simulink model "Dc_shunt_motor_model_not_verified"  (R2021b)
settings: Solver=VariableStepAuto  StartTime=0.0  StopTime=10.0  RelTol=1e-3
settings Model: Creator=victor  LastModifiedBy=victor

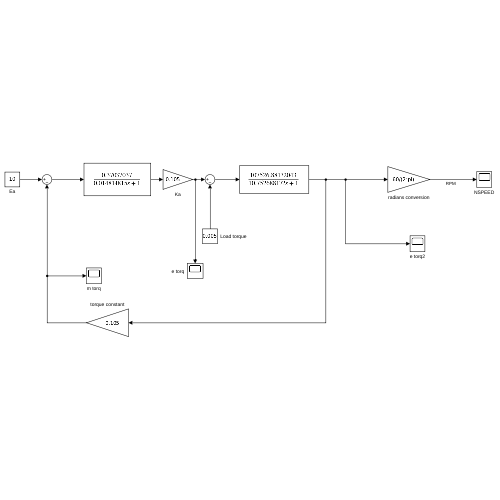
[thumbnail: Simulink's stored preview of the top-level diagram]
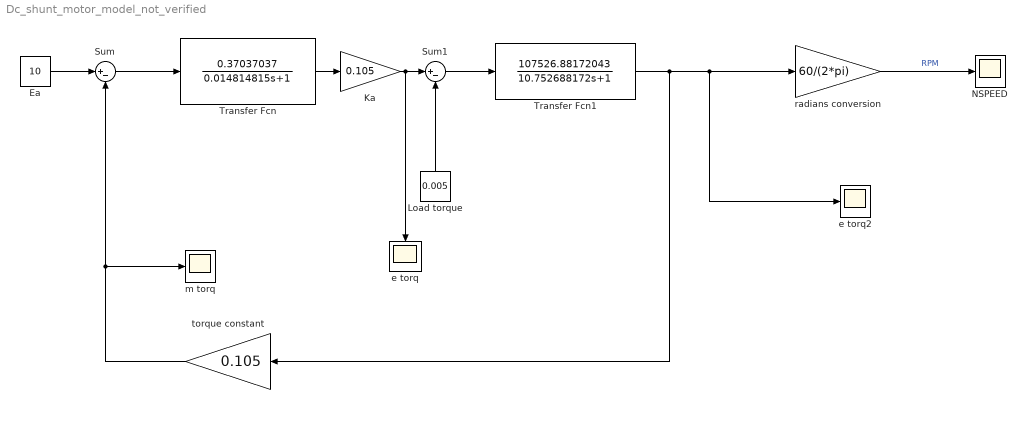
== system Dc_shunt_motor_model_not_verified ==
  Ea : Constant  Value=10
  Ka : Gain  Gain=0.105
  Load torque : Constant  Value=0.005
  NSPEED : Scope
  Sum : Sum  Inputs=|+-
  Sum1 : Sum  Inputs=|+-
  Transfer Fcn : TransferFcn  Numerator=[0.37037037]  Denominator=[0.014814815 1]
  Transfer Fcn1 : TransferFcn  Numerator=[107526.88172043]  Denominator=[10.752688172 1]
  e torq : Scope
  e torq2 : Scope
  m torq : Scope
  radians conversion : Gain  Gain=60/(2*pi)
  torque constant : Gain  Gain=0.105
  wires:
  torque constant/1 -> Sum/2, m torq/1
  Transfer Fcn/1 -> Ka/1
  Sum/1 -> Transfer Fcn/1
  Ka/1 -> e torq/1, Sum1/1
  Sum1/1 -> Transfer Fcn1/1
  Transfer Fcn1/1 -> torque constant/1, e torq2/1, radians conversion/1
  Load torque/1 -> Sum1/2
  radians conversion/1 -> NSPEED/1  "RPM"
  Ea/1 -> Sum/1
